simulink model "Example_6"  (R2020a)
settings: Solver=VariableStepAuto  StartTime=0.0  StopTime=10.0  RelTol=1e-3
libraries: simulink x2
settings Model: Creator=Kundan Patil  LastModifiedBy=Kundan Patil

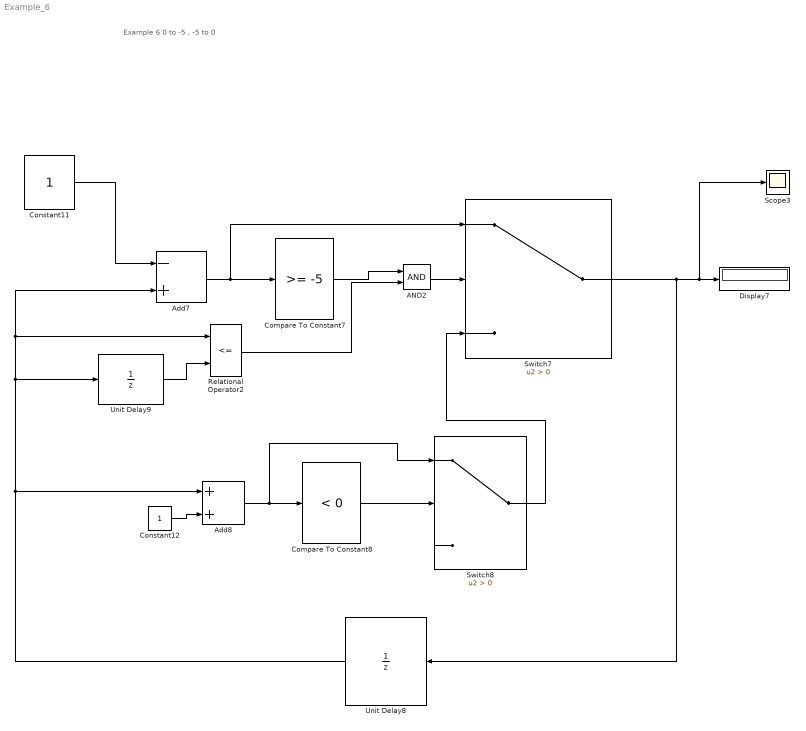
== system Example_6 ==
  note: Example 6
      | 0 to -5 , -5 to 0
  AND2 : Logic  AllPortsSameDT=off  OutDataTypeStr=boolean
  Add7 : Sum  Inputs=-+
  Add8 : Sum
  Compare To Constant7 : simulink/Logic and Bit Operations/Compare To Constant  relop=>=  const=-5  OutDataTypeStr=boolean
  Compare To Constant8 : simulink/Logic and Bit Operations/Compare To Constant  relop=<  const=0  OutDataTypeStr=boolean
  Constant11 : Constant
  Constant12 : Constant
  Display7 : Display
  Relational Operator2 : RelationalOperator  Operator=<=  OutDataTypeStr=boolean  RndMeth=Simplest
  Scope3 : Scope
  Switch7 : Switch  Criteria=u2 > Threshold
  Switch8 : Switch  Criteria=u2 > Threshold
  Unit Delay8 : UnitDelay  InitialCondition=1  SampleTime=-1  HasFrameUpgradeWarning=on
  Unit Delay9 : UnitDelay  InitialCondition=1  SampleTime=-1  HasFrameUpgradeWarning=on
  wires:
  Constant12/1 -> Add8/2
  AND2/1 -> Switch7/2
  Constant11/1 -> Add7/1
  Relational Operator2/1 -> AND2/2
  Compare To Constant8/1 -> Switch8/2
  Add8/1 -> Switch8/1, Compare To Constant8/1
  Switch7/1 -> Unit Delay8/1, Scope3/1, Display7/1
  Unit Delay8/1 -> Add7/2, Relational Operator2/1, Unit Delay9/1, Add8/1
  Unit Delay9/1 -> Relational Operator2/2
  Switch8/1 -> Switch7/3
  Compare To Constant7/1 -> AND2/1
  Add7/1 -> Switch7/1, Compare To Constant7/1
